simulink library "pixhawk_slib_swarm"  (R2022b)
settings: Solver=ode45  StartTime=0.0  StopTime=10.0  RelTol=1e-3
libraries: $bdroot x3, etargetslib x2, simulink x2
(part 1 of 2)
settings Model: Creator=skuznick  LastModifiedBy=童俊豪
settings SolverCC: AlgebraicLoopSolver=TrustRegion
settings DataIOCC: LimitDataPoints=on  SaveFormat=Array  ReturnWorkspaceOutputs=off
settings OptimizationCC: BlockReduction=off  BooleanDataType=off  LifeSpan=inf
settings DebuggingCC: SaveWithParameterizedLinksMsg=none  UnderspecifiedInitializationDetection=Classic  MergeDetectMultiDrivingBlocksExec=none  SignalResolutionControl=TryResolveAllWithWarning  UnconnectedInputMsg=warning  UnconnectedOutputMsg=warning  UnconnectedLineMsg=warning  AllowSymbolicDim=off  SFUnexpectedBacktrackingDiag=warning  SFNoUnconditionalDefaultTransitionDiag=warning  SFExecutionAtInitializationDiag=none  SFMachineParentedDataDiag=warning  ArithmeticOperatorsInVariantConditions=warning
settings HardwareCC: ProdBitPerPointer=32  ProdBitPerSizeT=32  ProdBitPerPtrDiffT=32  ProdLargestAtomicFloat=None  ProdIntDivRoundTo=Undefined  ProdEndianess=Unspecified  ProdWordSize=32  ProdHWDeviceType=32-bit Generic  TargetUnknown=on
settings ModelReferenceCC: EnableRefExpFcnMdlSchedulingChecks=on  PropagateSignalLabelsOutOfModel=off
settings SFSimCC: SimUseLocalCustomCode=off  CustomCodeUndefinedFunction=UseInterfaceOnly
settings RTWCC: RTWUseLocalCustomCode=off
settings CodeAppCC: StateflowObjectComments=on
settings GRTTargetCC: TargetLangStandard=C89/C90 (ANSI)
settings ConfigComp: CovMetricSettings=dw  CovSaveCumulativeToWorkspaceVar=on  CovSaveSingleToWorkspaceVar=on  CovExternalEMLEnable=off  CovSFcnEnable=off

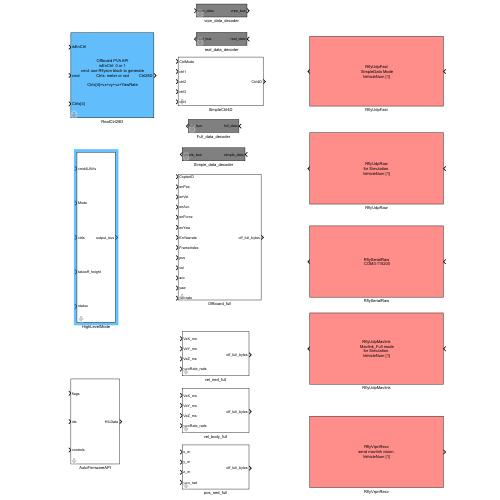
[thumbnail: Simulink's stored preview of the top-level diagram]
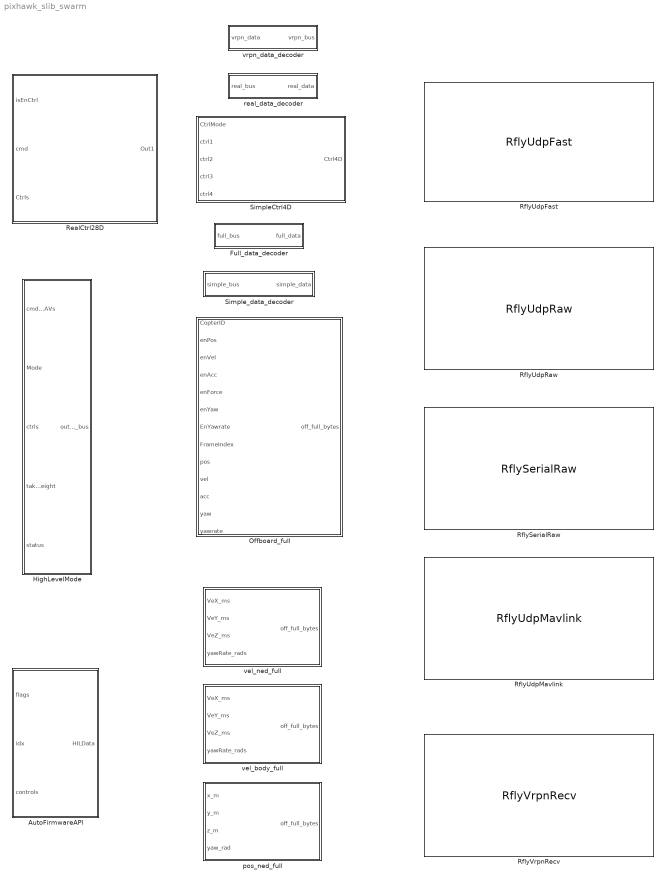
== system pixhawk_slib_swarm ==
  AutoFirmwareAPI : Subsystem  mask(AutoFirmwareAPI){}
      mask help:
      | This model is designed to generate 28 dims data for uav control with auto generated PX4  firmware by MATLAB.
      | The input data is to describe hil_actuator_controls, which has following meanings:
      | flags--user defined,  just keep sending and parsing consistent.
      | idx--for support more information, idx=0, treated as rfly_ctrl; idx=1, treated as rfly_ctrl1;idx=2, treated as rfly_ctrl2.
      | controls--detail imformation,can be control law or obstacle imformation.
      mask Help: eval('sharedhelp(''AutoFirmwareAPI'')');
  Full_data_decoder : Subsystem
      mask Help: eval('sharedhelp(''Full_data_decoder'')');
      mask DialogControl Control2 Prompt: (Add text here)
  HighLevelMode : Subsystem
      mask help:
      | Mode Control.
      |
      | 1 cmdUAVs should generate by "offical RflySim team" cmdUAVs "Rotary Switch".
      | 2   Mode will be explained as follows:
      |     Mode==1, x+y+z+yaw
      |     Mode==2, vx+vy+vz+yawrate
      |     Mode==3, accx+accy+accz+yawrate
      |     others, not supported
      | 3 ctrls only use first 4 elements and is described in local NED frame.
      | 4 takeoff_height, takeoff height.
      | 5 status means whether self check is passed, if not use, set true. Nothing will be send when status==false.
      mask Help: eval('sharedhelp(''HighLevelMode'')');
  Offboard_full : Subsystem
      mask Help: eval('sharedhelp(''Offboard_full'')');
      mask DialogControl Control2 Prompt: (Add text here)
  RealCtrl28D : Subsystem  mask{isX=off, isY=off, isZ=off, isVx=on, isVy=on, isVz=on, isAx=off, isAy=off, isAz=off, isYaw=off, isYawRate=on, EnIdxList=[1], isRcc=off, isForce=off, SamTime=-1}
      mask prompts: isX "x"; isY "y"; isZ "z"; isVx "vx"; isVy "vy"; isVz "vz"; isAx "ax"; isAy "ay"; isAz "az"; isYaw "yaw"; isYawRate "yawrate"; EnIdxList "mapList"; isRcc "Simulate Rcc Direct"; isForce "Enable Force"; SamTime "Sample Time (s)"
      mask help:
      | You can check the channels and prepare an input signal Ctrls with dimension and sequence corresponding to the of the checked channels.
      |
      | This Block enable offboard control for x y z vx vy vz ax ay az yaw yawrate，and support simulated Rcc direct control.
      |
      | # NED local world frame
      | x,y,z: position # in meters
      | Vx,Vy,Vz: velocity # in meters/second
      | Ax,Ay,Az: acceleration # in meters/second^2
      | yaw: euler angle of desired attitude in radians -PI..+PI
      | yawspeed: angular velocity around NED frame z-axis in radians/second
      |
      | In configuration page:
      | If "Simulate Rcc Direct" is checked, the module will send rcc signals to vehicle,  with relationship [vx, vy, vz, yawrate]->[ch1, ch2, ch3, ch4]. The user's [vx, vy, vz, yawrate] just in range [-1, 1], the block will map it to [1000-2000] automatically.
      | If "Enable Force" is checked, [ax, ay, az] will be treated as force.
      mask init:
      | SamTime=double(SamTime);
      mask Help: eval('sharedhelp(''RealCtrl28D'')');
      mask DialogControl Control2 Prompt: Select channels to control
      mask DialogControl Container3 Prompt: Option Functions
      mask Display:
      | nameList=["x";"y";"z";"vx";"vy";"vz";"ax";"ay";"az";"Yaw";"YawRate"];
      | nameList2=["isX";"isY";"isZ";"isVx";"isVy";"isVz";"isAx";"isAy";"isAz";"isYaw";"isYawRate"];
      | 
      | idx=0;
      | DispName='';
      | for i=1:length(nameList2)
      |     str0=char(nameList2(i));
      |     if strcmp(get_param(gcb,str0),'on') == true
      |         idx=idx+1;
      |         if idx==1
      |             DispName=[DispName,'',char(nameList(i))];
      |         else
      |             DispName=[DispName,'+',char(nameList(i))];
      |         end
      | 
      |         if mod(idx,4)==0
      |             DispName=[DispName,'\n'];
      |         end
      |     end
      | end
      | 
      | 
      | port_label('input', 1, 'isEnCtrl');
      | port_label('input', 2, 'cmd');
      | port_label('input', 3, ['Ctrls[',num2str(idx),']']);
      | port_label('output', 1, 'Ctrl28D');
      | 
      | fprintf(['Offboard PVA API\n isEnCtrl: 0 or 1 \n cmd: use Rflysim block to generate \n Ctrls: meter or rad \n\n','Ctrls[',num2str(idx),']=',DispName]);
      | 
      | set_param([gcb,'/isEnCtrl'],'PortDimensions',num2str(1));
      | set_param([gcb,'/cmd'],'PortDimensions',num2str(1));
      | set_param([gcb,'/Ctrls'],'PortDimensions',num2str(idx));
      | %set_param([gcb,'/OffboardAdvCtrlAPI'],'PortDimensions',num2str(idx));
  RflySerialRaw : S-Function  FunctionName=RflySerialRaw  Parameters=portname,baud,T  SFunctionDeploymentMode=off  EnableBusSupport=off  mask(RflySerialFast API){portname=COM3, baud=115200, T=1/30}
      mask prompts: portname "SerialPortName:"; baud "Baudrate or list (e.g., [57600,115200])"; T "Sample Time"
      mask help:
      | This block receives bytes from an serial connection.
      | 1. SerialPortName: Input the name of one pixhawk COM or multiple pixhawk COMs seperated by ','. For example, COM3 or COM3,COM4,COM5
      | 2. SelectAvailablePort: Prompt a window to select one or multiple COM port name
      | 3. baudrate or list: input the buadrate of all COMs or use a list to specify baudrate of each COM.
      |
      | input&output: variable-length unit_8 vector data from or to serial buffer.
      mask init:
      | if strcmp(computer(), 'PCWIN64')
      |     if isnumeric(portname)
      |         if portname>=10
      |             portname=['\\.\COM'+num2str(portname)];
      |         else
      |             portname=['COM'+num2str(portname)];
      |         end
      |     else
      |         dd=strsplit(portname,',');
      |         namestr='';
      |         for i=1:length(dd)
      |             name=strtrim(dd{1,i});
      |             if ~isempty(str2num(name))
      |                 nNnum=str2double(name);
      |                 if nNnum>=10
      |                     name=['\\.\COM'+num2str(nNnum)];
      |                 else
      |                     name=['COM'+num2str(nNnum)];
      |                 end
      |             end
      |             
      |         
      |             if length(name)>4
      |                 name=['\\.\',name];
      |             end
      |         
      |             namestr=[namestr,name];
      |             if i~=length(dd)
      |                 namestr=[namestr,','];
      |             end
      |         end
      |         portname=namestr;
      |     end
      | end
      mask Help: eval('sharedhelp(''RflySerialRaw'')');
      mask DialogControl Control3 Prompt: SelectAvailablePort
      mask DialogControl Control3 Callback:
      | portList = seriallist;
      | if ~isempty(portList)
      |     CellTmp={};
      |     for i=1:length(portList)
      |         CellTmp{i,1}=char(portList(i));
      |     end
      |     [indx,tf] = listdlg('ListString',CellTmp,'ListSize',[160,100]);
      |     if tf
      |         maskObj = Simulink.Mask.get(gcb);
      |         for i=1:length(maskObj.Parameters)
      |             if strcmp(maskObj.Parameters(i).Name,'portname')
      |                 myStr='';
      |                 for j=1:length(indx)
      |                     myStr=[myStr,CellTmp{indx(j),1}];
      |                     if j~=length(indx)
      |                         myStr=[myStr,','];
      |                     end
      |                 end
      |                 %maskObj.Parameters(i).set('Value',myStr);
      |                 maskObj.Parameters(i).Value=myStr;
      |             end
      |         end
      | 
      |     end
      | else
      |     msgbox('No avaliable COM port.')
      | end
      mask Display: fprintf(['RflySerialRaw\n ',get_param(gcb,'portname'),':',get_param(gcb,'baud')]);
  RflyUdpFast : S-Function  FunctionName=RflyUdpFast  Parameters=idx,num,modeValue,T,ip,Gps,port,isSame  SFunctionDeploymentMode=off  EnableBusSupport=off  mask(RflyUdpFast API){ip=127.0.0.1, idx=1, num=1, mode=SimpleData Mode, Gps=[40.1540302,116.2593683,50.0], port=20100, isSame=off, T=1/30, modeValue=0}
      mask prompts: ip "Target IP Address"; idx "Start CopterID"; num "Vehicle number or CopterID list (e.g., [1 3 4])"; mode "UDP Mode"; Gps "GPS Orin [Lat Lon (degree) Alt(m)] for GlobalPos"; port "Base UDP Port (for CopterID#1)"; isSame "useSamePort"; T "Sample Time"
      mask help:
      | RflySimAPIs for multiple uav data acquire and control
      | 1. Target IP: The IP of PC running CopterSims to receive data
      | 2. Vehicle number: Total vehicle number with StartID=1.
      | For example Vehicle number=3 for a CopterID list [1 2 3]
      | 3. CopterID List: a vector of CopterIDs, like [1 2 3] or [1:3] or [4 5 7]
      | 4. UDP Mode: Full or simple mode to transmit data
      | 5. GPS Orin: the lat lon alt of GPS position for calculate global position
      | 6. check the "Help" button for the definition
      mask init:
      | if strcmp(mode,'FullData Mode')
      |     modeValue = 0;
      | elseif strcmp(mode,'SimpleData Mode') 
      |     modeValue = 1;
      | elseif strcmp(mode,'UltraSimple Mode') 
      |     modeValue = 2;
      | else
      |     modeValue = 0;
      | end
      | 
      | if length(num)==1
      |     if str2double(get_param(gcb,'num')) == num
      |         num = 1:num;
      |     end
      | end
      mask Help: eval('sharedhelp(''RflyUdpFast'')');
      mask TypeOptions mode: FullData Mode | SimpleData Mode
      mask Display:
      | numstr=get_param(gcb,'num');
      | if strcmp(numstr,'1')
      |     numstr='[1]';
      | end
      | fprintf(['RflyUdpFast\n ',get_param(gcb,'mode'),'\nVehicleNum ',numstr]);
  RflyUdpMavlink : S-Function  FunctionName=RflyUdpMavlink  Parameters=idx,num,ip,T,port,isSame,Gps,udpmode  SFunctionDeploymentMode=off  EnableBusSupport=off  mask(RflyUdpReal API){idx=1, ip1=127.0.0.1, ip=192.168.31.101, num=1, port=15501, Gps=[40.1540302,116.2593683,50.0], udpmode=Mavlink_Full, T=1/30, isSame=off}
      mask prompts: idx "Start Index"; ip1 "Target IP Address"; ip "Base IP Address or IP list seperated by ','"; num "Vehicle number or CopterID list (e.g., [1 3 4])"; port "Base UDP Port or list"; Gps "GPS Orin [Lat Lon (degree) Alt(m)] for GlobalPos"; udpmode "Udp Mode"; T "Sample Time"; isSame "RealflyMode"
      mask help:
      | RflySimAPIs for multiple real uav data acquire and control
      | 1. Base IP: The bash IP of the first UAV to receive MAVLink data
      | 2. IP list: a string like 191.168.151.101,191.168.151.102 to specify the ip of each UAV
      | 3. Vehicle number: Total vehicle number with StartID=1.
      | For example Vehicle number=3 for a CopterID list [1 2 3]
      | 4. CopterID List: a vector of CopterIDs, like [1 2 3] or [1:3] or [4 5 7]
      | 5. Base UDP Port: The base port of the first UAV's mavlink port. You can also use a port list to specify the port of each UAV
      | 6. RealflyMode: Checked for real uav control, the IP and port will auto increase 1 according to CopterID increase.
      | Not checked for RflySim UDP simulation, the IP will not change and the port will +2 for each CopterID.
      |
      | Input and output char arrays from buf for mavlink encode and decoder
      mask init:
      | if isSame<0.5
      |     ip=ip1;
      | end
      | 
      | if length(num)==1
      |     if str2double(get_param(gcb,'num')) == num
      |         num = 1:num;
      |     end
      | end
      mask Help: eval('sharedhelp(''RflyUdpMavlink'')');
      mask TypeOptions udpmode: Mavlink_Full | Mavlink_Simp | Mavlink_Real
      mask Callback isSame:
      | maskObj = Simulink.Mask.get(gcb);
      | for i=1:length(maskObj.Parameters)
      |     if strcmp(maskObj.Parameters(i).Name,'Gps')
      |         if strcmp(get_param(gcb,'isSame'),'off')
      |             if strcmp(maskObj.Parameters(i).Enabled,'off')
      |                 maskObj.Parameters(i).Enabled='on';
      |                 maskObj.Parameters(i).Visible='on';
      |             end
      |         else
      |             if strcmp(maskObj.Parameters(i).Enabled,'on')
      |                 maskObj.Parameters(i).Enabled='off';
      |                 maskObj.Parameters(i).Visible='off';
      |             end
      |         end
      |     end
      | end
      | for i=1:length(maskObj.Parameters)
      |     if strcmp(maskObj.Parameters(i).Name,'port')
      |         if strcmp(get_param(gcb,'isSame'),'off')
      |             if strcmp(maskObj.Parameters(i).Enabled,'on')
      |                 maskObj.Parameters(i).Enabled='off';
      |                 maskObj.Parameters(i).Visible='off';
      |             end
      |         else
      |             if strcmp(maskObj.Parameters(i).Enabled,'off')
      |                 maskObj.Parameters(i).Enabled='on';
      |                 maskObj.Parameters(i).Visible='on';
      |             end
      |         end
      |     end
      | end
      | for i=1:length(maskObj.Parameters)
      |     if strcmp(maskObj.Parameters(i).Name,'ip1')
      |         if strcmp(get_param(gcb,'isSame'),'on')
      |             if strcmp(maskObj.Parameters(i).Enabled,'on')
      |                 maskObj.Parameters(i).Enabled='off';
      |                 maskObj.Parameters(i).Visible='off';
      |             end
      |         else
      |             if strcmp(maskObj.Parameters(i).Enabled,'off')
      |                 maskObj.Parameters(i).Enabled='on';
      |                 maskObj.Parameters(i).Visible='on';
      |             end
      |         end
      |     end
      | end
      | for i=1:length(maskObj.Parameters)
      |     if strcmp(maskObj.Parameters(i).Name,'ip')
      |         if strcmp(get_param(gcb,'isSame'),'on')
      |             if strcmp(maskObj.Parameters(i).Enabled,'off')
      |                 maskObj.Parameters(i).Enabled='on';
      |                 maskObj.Parameters(i).Visible='on';
      |             end
      |         else
      |             if strcmp(maskObj.Parameters(i).Enabled,'on')
      |                 maskObj.Parameters(i).Enabled='off';
      |                 maskObj.Parameters(i).Visible='off';
      |             end
      |         end
      |     end
      | end
      | 
      | for i=1:length(maskObj.Parameters)
      |     if strcmp(maskObj.Parameters(i).Name,'udpmode')
      |         if strcmp(get_param(gcb,'isSame'),'off')
      |             if strcmp(maskObj.Parameters(i).Enabled,'off')
      |                 maskObj.Parameters(i).Enabled='on';
      |                 maskObj.Parameters(i).Visible='on';
      |             end
      |         else
      |             if strcmp(maskObj.Parameters(i).Enabled,'on')
      |                 maskObj.Parameters(i).Enabled='off';
      |                 maskObj.Parameters(i).Visible='off';
      |             end
      |         end
      |     end
      | end
      mask Display:
      | myname='for Simulation.';
      | if strcmp(get_param(gcb,'isSame'),'on')
      |     myname='for Real fly.';
      | end
      | numstr=get_param(gcb,'num');
      | if strcmp(numstr,'1')
      |     numstr='[1]';
      | end
      | fprintf(['RflyUdpMavlink\n ',get_param(gcb,'udpmode'),' mode\n',myname,'\nVehicleNum ',numstr]);
  RflyUdpRaw : S-Function  FunctionName=RflyUdpRaw  Parameters=idx,num,ip,T,port,isSame  SFunctionDeploymentMode=off  EnableBusSupport=off  mask(RflyUdpReal API){idx=1, ip1=127.0.0.1, ip=192.168.31.101, num=1, port=15501, T=1/30, isSame=off}
      mask prompts: idx "Start Index"; ip1 "Target IP Address"; ip "Base IP Address or IP list seperated by ','"; num "Vehicle number or CopterID list (e.g., [1 3 4])"; port "Base UDP Port or list"; T "Sample Time"; isSame "RealflyMode"
      mask help:
      | RflySimAPIs for multiple real uav data acquire and control
      | 1. IP Address: The bash IP of the first UAV to receive MAVLink data (127.0.0.1 for Simulation or remote ip for real fly)
      | 2. IP list: a string like 191.168.151.101,191.168.151.102 to specify the ip of each UAV
      | 3. Vehicle number: Total vehicle number with StartID=1.
      | For example Vehicle number=3 for a CopterID list [1 2 3]
      | 4. CopterID List: a vector of CopterIDs, like [1 2 3] or [1:3] or [4 5 7]
      | 5. Base UDP Port: The base port of the first UAV's mavlink port. You can also use a port list to specify the port of each UAV
      | 6. RealflyMode: Checked for real uav control, the IP and port will auto increase 1 according to CopterID increase.
      | Not checked for RflySim UDP simulation, the IP will not change and the port will +2 for each CopterID.
      |
      | Input and output char arrays from buf for mavlink encode and decoder
      mask init:
      | if isSame<0.5
      |     ip=ip1;
      | end
      | 
      | if length(num)==1
      |     if str2double(get_param(gcb,'num')) == num
      |         num = 1:num;
      |     end
      | end
      mask Help: eval('sharedhelp(''RflyUdpRaw'')');
      mask Callback isSame:
      | maskObj = Simulink.Mask.get(gcb);
      | for i=1:length(maskObj.Parameters)
      |     if strcmp(maskObj.Parameters(i).Name,'port')
      |         if strcmp(get_param(gcb,'isSame'),'off')
      |             maskObj.Parameters(i).Enabled='off';
      |             maskObj.Parameters(i).Visible='off';
      |         else
      |             maskObj.Parameters(i).Enabled='on';
      |             maskObj.Parameters(i).Visible='on';
      |         end
      |     end
      | end
      | for i=1:length(maskObj.Parameters)
      |     if strcmp(maskObj.Parameters(i).Name,'ip1')
      |         if strcmp(get_param(gcb,'isSame'),'on')
      |             maskObj.Parameters(i).Enabled='off';
      |             maskObj.Parameters(i).Visible='off';
      |         else
      |             maskObj.Parameters(i).Enabled='on';
      |             maskObj.Parameters(i).Visible='on';
      |         end
      |     end
      | end
      | for i=1:length(maskObj.Parameters)
      |     if strcmp(maskObj.Parameters(i).Name,'ip')
      |         if strcmp(get_param(gcb,'isSame'),'on')
      |             maskObj.Parameters(i).Enabled='on';
      |             maskObj.Parameters(i).Visible='on';
      |         else
      |             maskObj.Parameters(i).Enabled='off';
      |             maskObj.Parameters(i).Visible='off';
      |         end
      |     end
      | end
      mask Display:
      | myname='for Simulation.';
      | if strcmp(get_param(gcb,'isSame'),'on')
      |     myname='for Real fly.';
      | end
      | numstr=get_param(gcb,'num');
      | if strcmp(numstr,'1')
      |     numstr='[1]';
      | end
      | fprintf(['RflyUdpRaw\n',myname,'\nVehicleNum ',numstr]);
  RflyVrpnRecv : S-Function  FunctionName=RflyVrpnRecv  Parameters=vrpn_ip,num,T,isSend,drone_ip,drone_port,vrScaleX,vrScaleY,vrScaleZ  SFunctionDeploymentMode=off  EnableBusSupport=off  mask(RflyUdpReal API){vrpn_ip=127.0.0.1, num=1, T=1/30, isSend=on, drone_ip=192.168.151.101, drone_port=15501, vrScaleX=1.0, vrScaleY=1.0, vrScaleZ=1.0}
      mask prompts: vrpn_ip "Vrpn IP Address"; num "Vehicle number or CopterID list (e.g., [1 3 4])"; T "Sample Time"; isSend "isSendVision"; drone_ip "Drone base IP Address or IP list seperated by ','"; drone_port "Drone base UDP Port or list"; vrScaleX "VR Scale X"; vrScaleY "Y"; vrScaleZ "Z"
      mask help:
      | RflySimAPIs for multiple real uav data acquire and control
      | 1. Base IP: The bash IP of the first UAV to receive MAVLink data
      | 2. IP list: a string like 191.168.151.101,191.168.151.102 to specify the ip of each UAV
      | 3. Vehicle number: Total vehicle number with StartID=1.
      | For example Vehicle number=3 for a CopterID list [1 2 3]
      | 4. CopterID List: a vector of CopterIDs, like [1 2 3] or [1:3] or [4 5 7]
      | 5. Base UDP Port: The base port of the first UAV's mavlink port. You can also use a port list to specify the port of each UAV
      | 6. RealflyMode: Checked for real uav control, the IP and port will auto increase 1 according to CopterID increase.
      | 7.Scale for combination of virtual and real elements for X direction.
      | 8.Scale for combination of virtual and real elements for Y direction.
      | 9.Scale for combination of virtual and real elements for vertical direction.
      | Not checked for RflySim UDP simulation, the IP will not change and the port will +2 for each CopterID.
      |
      | Input and output char arrays from buf for mavlink encode and decoder
      mask init:
      | if length(num)==1
      |     if str2double(get_param(gcb,'num')) == num
      |         num = 1:num;
      |     end
      | end
      mask Help: eval('sharedhelp(''RflyVrpnRecv'')');
      mask Callback isSend:
      | maskObj = Simulink.Mask.get(gcb);
      | for i=1:length(maskObj.Parameters)
      |     if strcmp(maskObj.Parameters(i).Name,'drone_ip')
      |         if strcmp(get_param(gcb,'isSend'),'on')
      |             if strcmp(maskObj.Parameters(i).Enabled,'off')
      |                 maskObj.Parameters(i).Enabled='on';
      |                 maskObj.Parameters(i).Visible='on';
      |             end
      |         else
      |             if strcmp(maskObj.Parameters(i).Enabled,'on')
      |                 maskObj.Parameters(i).Enabled='off';
      |                 maskObj.Parameters(i).Visible='off';
      |             end
      |         end
      |     end
      | end
      | for i=1:length(maskObj.Parameters)
      |     if strcmp(maskObj.Parameters(i).Name,'drone_port')
      |         if strcmp(get_param(gcb,'isSend'),'on')
      |             if strcmp(maskObj.Parameters(i).Enabled,'off')
      |                 maskObj.Parameters(i).Enabled='on';
      |                 maskObj.Parameters(i).Visible='on';
      |             end
      |         else
      |             if strcmp(maskObj.Parameters(i).Enabled,'on')
      |                 maskObj.Parameters(i).Enabled='off';
      |                 maskObj.Parameters(i).Visible='off';
      |             end
      |         end
      |     end
      | end
      mask Display:
      | myname='not send vision.';
      | if strcmp(get_param(gcb,'isSend'),'on')
      |     myname='send mavlink vision.';
      | end
      | numstr=get_param(gcb,'num');
      | if strcmp(numstr,'1')
      |     numstr='[1]';
      | end
      | fprintf(['RflyVrpnRecv\n',myname,'\nVehicleNum ',numstr]);
  SimpleCtrl4D : Subsystem
      mask Help: eval('sharedhelp(''SimpleCtrl4D'')');
      mask DialogControl Control2 Prompt: (Add text here)
  Simple_data_decoder : Subsystem
      mask Help: eval('sharedhelp(''Simple_data_decoder'')');
      mask DialogControl Control2 Prompt: (Add text here)
  pos_ned_full : Subsystem
      mask Help: eval('sharedhelp(''pos_ned_full'')');
      mask DialogControl Control2 Prompt: (Add text here)
  real_data_decoder : Subsystem
      mask Help: eval('sharedhelp(''real_data_decoder'')');
      mask DialogControl Control2 Prompt: (Add text here)
  vel_body_full : Subsystem
      mask Help: eval('sharedhelp(''vel_body_full'')');
      mask DialogControl Control2 Prompt: (Add text here)
  vel_ned_full : Subsystem
      mask Help: eval('sharedhelp(''vel_ned_full'')');
      mask DialogControl Control2 Prompt: (Add text here)
  vrpn_data_decoder : Subsystem
      mask Help: eval('sharedhelp(''vrpn_data_decoder'')');
      mask DialogControl Control2 Prompt: (Add text here)

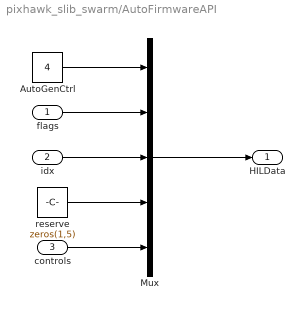
== system pixhawk_slib_swarm/AutoFirmwareAPI ==
  flags : Inport
  idx : Inport  Port=2
  controls : Inport  Port=3
  AutoGenCtrl : Constant  Value=4
  Mux : Mux  Inputs=5
  reserve : Constant  Value=zeros(1,5)
  HILData : Outport  VectorParamsAs1DForOutWhenUnconnected=off
  wires:
  Mux/1 -> HILData/1
  flags/1 -> Mux/2
  idx/1 -> Mux/3
  controls/1 -> Mux/5
  AutoGenCtrl/1 -> Mux/1
  reserve/1 -> Mux/4

== system pixhawk_slib_swarm/Full_data_decoder ==
  note: AngEular
  note: localVel
  note: localPos
  full_data : Inport
  Bus Creator : BusCreator  Inputs=17
  Decoder1 : MATLAB Function  TreatAsAtomicUnit=on
  full_bus : Outport  VectorParamsAs1DForOutWhenUnconnected=off
  wires:
  Decoder1/17(resrveFloat) -> Bus Creator/17  "resrveFloat"
  Decoder1/1(globalPos) -> Bus Creator/1  "globalPos"
  Decoder1/7(gpsHome) -> Bus Creator/7  "gpsHome"
  Decoder1/12(satellites_visible) -> Bus Creator/12  "satellites_visible"
  Bus Creator/1 -> full_bus/1
  full_data/1 -> Decoder1/1(u)
  Decoder1/14(resrveInit) -> Bus Creator/14  "resrveInit"
  Decoder1/13(fix_type) -> Bus Creator/13  "fix_type"
  Decoder1/15(pos_horiz_accuracy) -> Bus Creator/15  "pos_horiz_accuracy"
  Decoder1/16(pos_vert_accuracy) -> Bus Creator/16
  Decoder1/9(copterID) -> Bus Creator/9  "copterID"
  Decoder1/10(relative_alt) -> Bus Creator/10  "relative_alt"
  Decoder1/11(hdg) -> Bus Creator/11  "hdg"
  Decoder1/8(time_boot_ms) -> Bus Creator/8  "time_boot_ms"
  Decoder1/6(GpsVel) -> Bus Creator/6  "GpsVel"
  Decoder1/5(GpsPos) -> Bus Creator/5  "GpsPos"
  Decoder1/2(AngEular) -> Bus Creator/2  "AngEular"
  Decoder1/3(localPos) -> Bus Creator/3  "localPos"
  Decoder1/4(localVel) -> Bus Creator/4  "localVel"

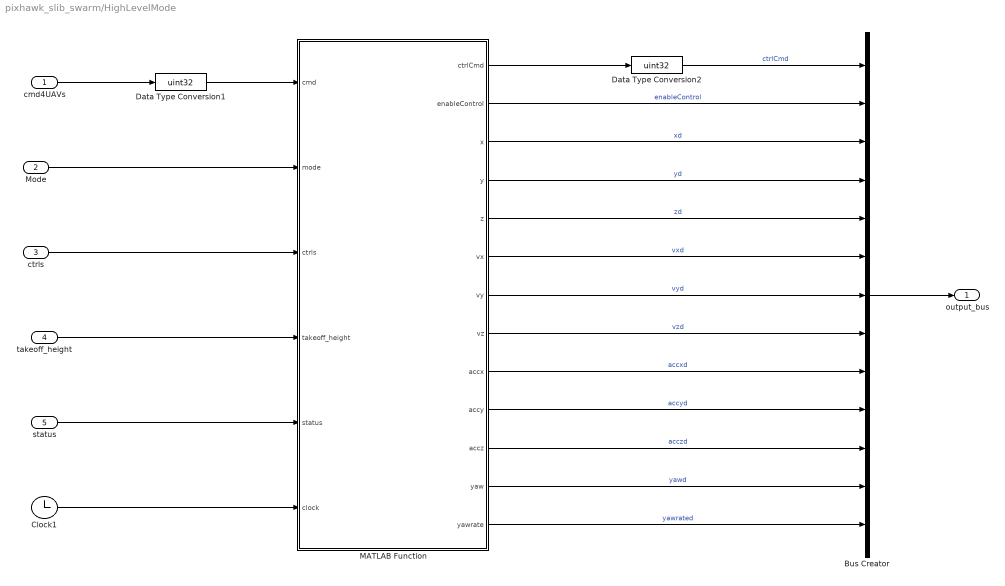
== system pixhawk_slib_swarm/HighLevelMode ==
  cmd4UAVs : Inport
  Mode : Inport  Port=2  PortDimensions=1
  ctrls : Inport  Port=3  PortDimensions=16
  takeoff_height : Inport  Port=4
  status : Inport  Port=5
  Bus Creator : BusCreator  Inputs=13
  Clock1 : Clock
  Data Type Conversion1 : DataTypeConversion  OutDataTypeStr=uint32  SaturateOnIntegerOverflow=off  RndMeth=Floor
  Data Type Conversion2 : DataTypeConversion  OutDataTypeStr=uint32  SaturateOnIntegerOverflow=off  RndMeth=Floor
  MATLAB Function : MATLAB Function  TreatAsAtomicUnit=on
  output_bus : Outport  VectorParamsAs1DForOutWhenUnconnected=off
  wires:
  cmd4UAVs/1 -> Data Type Conversion1/1
  Data Type Conversion1/1 -> MATLAB Function/1(cmd)
  Clock1/1 -> MATLAB Function/6(clock)
  status/1 -> MATLAB Function/5(status)
  MATLAB Function/1(ctrlCmd) -> Data Type Conversion2/1
  Data Type Conversion2/1 -> Bus Creator/1  "ctrlCmd"
  MATLAB Function/2(enableControl) -> Bus Creator/2  "enableControl"
  MATLAB Function/3(x) -> Bus Creator/3  "xd"
  MATLAB Function/4(y) -> Bus Creator/4  "yd"
  MATLAB Function/5(z) -> Bus Creator/5  "zd"
  MATLAB Function/6(vx) -> Bus Creator/6  "vxd"
  MATLAB Function/7(vy) -> Bus Creator/7  "vyd"
  MATLAB Function/8(vz) -> Bus Creator/8  "vzd"
  MATLAB Function/9(accx) -> Bus Creator/9  "accxd"
  MATLAB Function/10(accy) -> Bus Creator/10  "accyd"
  MATLAB Function/11(accz) -> Bus Creator/11  "acczd"
  MATLAB Function/12(yaw) -> Bus Creator/12  "yawd"
  MATLAB Function/13(yawrate) -> Bus Creator/13  "yawrated"
  ctrls/1 -> MATLAB Function/3(ctrls)
  Mode/1 -> MATLAB Function/2(mode)
  Bus Creator/1 -> output_bus/1
  takeoff_height/1 -> MATLAB Function/4(takeoff_height)

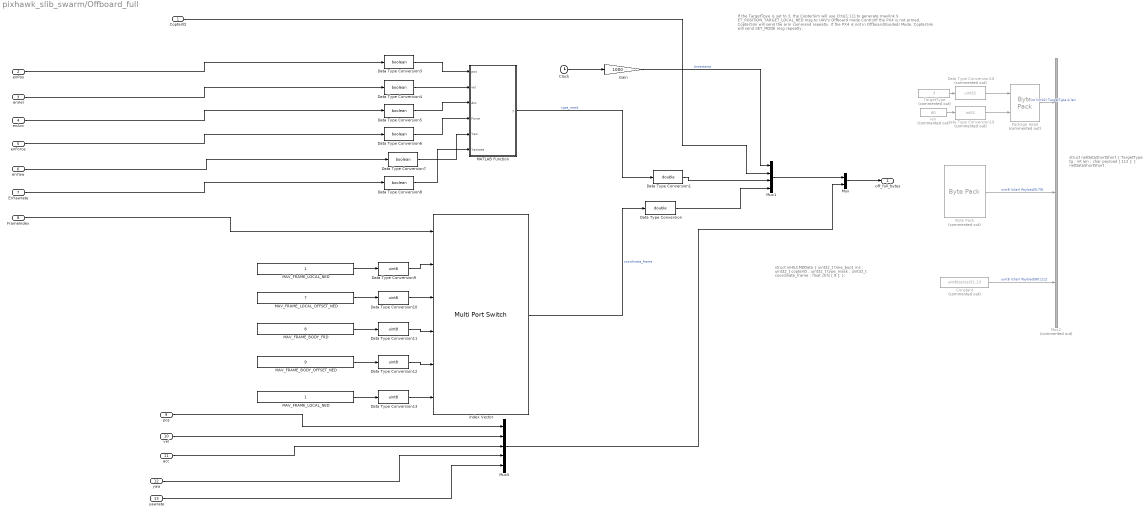
== system pixhawk_slib_swarm/Offboard_full ==
  note: struct netDataShortShort {
      | TargetType tg ;
      | int len ;
      | char payload [ 112 ];
      | } netDataShortShort ;
  note: struct inHILCMDData {
      | uint32_t time_boot_ms ;
      | uint32_t copterID ;
      | uint32_t type_mask ;
      | uint32_t coordinate_frame ;
      | float ctrls [ 9 ];
      | };
  note: If the TargetTpye is set to 3, the CopterSim will use Ctrs[1:11] to generate mavlink S ET_POSITION_TARGET_LOCAL_NED msg to UAV's Offboard mode Control，
      | If the PX4 is not armed, CopterSim will send the arm command repeatly. If the PX4 is not in Offboard(Guided) Mode, CopterSim will send SET_MODE msg repeatly.
  CopterID : Inport
  enPos : Inport  Port=2
  enVel : Inport  Port=3
  enAcc : Inport  Port=4
  enForce : Inport  Port=5
  enYaw : Inport  Port=6
  EnYawrate : Inport  Port=7
  FrameIndex : Inport  Port=8
  pos : Inport  Port=9  PortDimensions=3
  vel : Inport  Port=10  PortDimensions=3
  acc : Inport  Port=11  PortDimensions=3
  yaw : Inport  Port=12  PortDimensions=1
  yawrate : Inport  Port=13  PortDimensions=1
  Byte Pack : etargetslib/Byte Pack  Commented=on  datatypes={'uint32','single'}  byteAlign=1
  Clock : Clock
  Constant : Constant  Commented=on  Value=uint8(zeros(32,1))
  Data Type Conversion : DataTypeConversion  OutDataTypeStr=double  SaturateOnIntegerOverflow=off  RndMeth=Floor
  Data Type Conversion1 : DataTypeConversion  OutDataTypeStr=double  SaturateOnIntegerOverflow=off  RndMeth=Floor
  Data Type Conversion{9..13} (5 alike) : DataTypeConversion  OutDataTypeStr=uint8  SaturateOnIntegerOverflow=off  RndMeth=Floor
  Data Type Conversion18 : DataTypeConversion  Commented=on  OutDataTypeStr=uint32  SaturateOnIntegerOverflow=off  RndMeth=Floor
  Data Type Conversion19 : DataTypeConversion  Commented=on  OutDataTypeStr=int32  SaturateOnIntegerOverflow=off  RndMeth=Floor
  Data Type Conversion{3..8} (6 alike) : DataTypeConversion  OutDataTypeStr=boolean  SaturateOnIntegerOverflow=off  RndMeth=Floor
  Gain : Gain  Gain=1000
  Index Vector : MultiPortSwitch  DataPortOrder=Zero-based contiguous  Inputs=5  zeroidx=on  SaturateOnIntegerOverflow=off  InputSameDT=off
  MATLAB Function : MATLAB Function  TreatAsAtomicUnit=on
  MAV_FRAME_BODY_FRD : Constant  Value=8
  "MAV_FRAME_BODY_OFFSET_NED " : Constant  Value=9
  MAV_FRAME_LOCAL_NED : Constant
  "MAV_FRAME_LOCAL_NED " : Constant
  MAV_FRAME_LOCAL_OFFSET_NED : Constant  Value=7
  Mux : Mux  Inputs=2
  Mux1 : Mux
  Mux2 : Mux  Commented=on  Inputs=3
  Mux5 : Mux  Inputs=5
  Package Head : etargetslib/Byte Pack  Commented=on  datatypes={'uint32','int32'}  byteAlign=4
  TargetType : Constant  Commented=on  Value=3  OutDataTypeStr=Inherit: Inherit via back propagation
  len : Constant  Commented=on  Value=80  OutDataTypeStr=Inherit: Inherit via back propagation
  off_full_bytes : Outport
  wires:
  Data Type Conversion7/1 -> MATLAB Function/5(Yaw)
  Data Type Conversion6/1 -> MATLAB Function/4(Force)
  vel/1 -> Mux5/2
  MAV_FRAME_BODY_FRD/1 -> Data Type Conversion11/1
  Data Type Conversion3/1 -> MATLAB Function/1(pos)
  Data Type Conversion5/1 -> MATLAB Function/3(Acc)
  Data Type Conversion4/1 -> MATLAB Function/2(vel)
  Data Type Conversion8/1 -> MATLAB Function/6(Yawrate)
  enAcc/1 -> Data Type Conversion5/1
  enYaw/1 -> Data Type Conversion7/1
  EnYawrate/1 -> Data Type Conversion8/1
  enForce/1 -> Data Type Conversion6/1
  "MAV_FRAME_LOCAL_NED "/1 -> Data Type Conversion9/1
  enPos/1 -> Data Type Conversion3/1
  Data Type Conversion9/1 -> Index Vector/2
  Data Type Conversion10/1 -> Index Vector/3
  Index Vector/1 -> Data Type Conversion/1  "coordinate_frame"
  Constant/1 -> Mux2/3  "uint8 (char) Payload[80:111]"
  Data Type Conversion18/1 -> Package Head/1
  Clock/1 -> Gain/1
  len/1 -> Data Type Conversion19/1
  Mux5/1 -> Mux/2
  MATLAB Function/1(y) -> Data Type Conversion1/1  "type_mask"
  Package Head/1 -> Mux2/1  "int (int32) TargetType & len"
  TargetType/1 -> Data Type Conversion18/1
  Gain/1 -> Mux1/1  "timestamp"
  Data Type Conversion19/1 -> Package Head/2
  pos/1 -> Mux5/1
  Byte Pack/1 -> Mux2/2  "uint8 (char) Payload[0:79]"
  Data Type Conversion13/1 -> Index Vector/6
  Data Type Conversion12/1 -> Index Vector/5
  acc/1 -> Mux5/3
  FrameIndex/1 -> Index Vector/1
  MAV_FRAME_LOCAL_NED/1 -> Data Type Conversion13/1
  MAV_FRAME_LOCAL_OFFSET_NED/1 -> Data Type Conversion10/1
  Data Type Conversion11/1 -> Index Vector/4
  "MAV_FRAME_BODY_OFFSET_NED "/1 -> Data Type Conversion12/1
  enVel/1 -> Data Type Conversion4/1
  yaw/1 -> Mux5/4
  yawrate/1 -> Mux5/5
  CopterID/1 -> Mux1/2
  Mux1/1 -> Mux/1
  Mux/1 -> off_full_bytes/1
  Data Type Conversion/1 -> Mux1/4
  Data Type Conversion1/1 -> Mux1/3

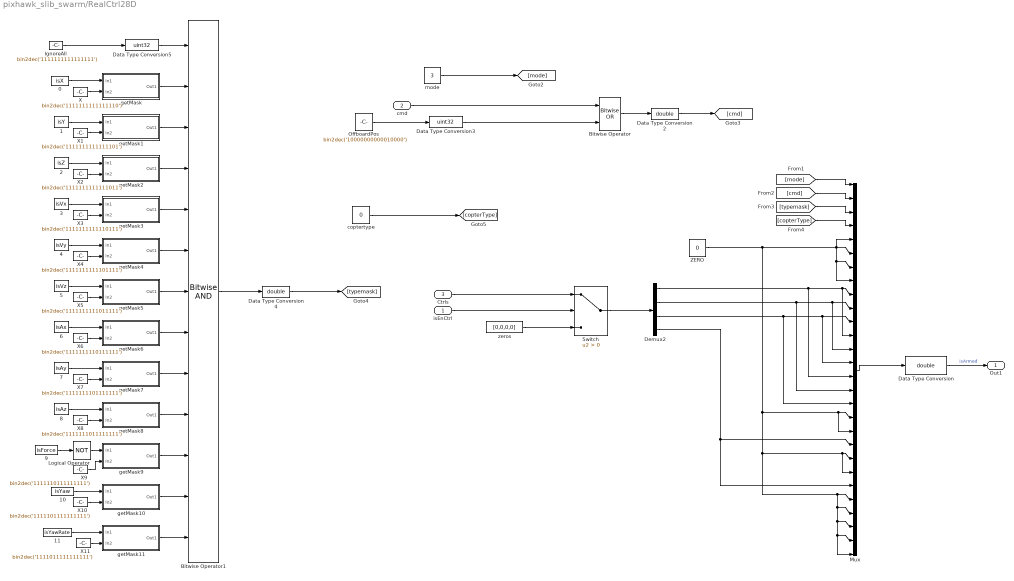
== system pixhawk_slib_swarm/RealCtrl28D ==
  isEnCtrl : Inport  PortDimensions=1
  cmd : Inport  Port=2  OutDataTypeStr=uint32  PortDimensions=1
  Ctrls : Inport  Port=3  PortDimensions=4
  0 : Constant  Value=isX
  1 : Constant  Value=isY
  10 : Constant  Value=isYaw
  11 : Constant  Value=isYawRate
  2 : Constant  Value=isZ
  3 : Constant  Value=isVx
  4 : Constant  Value=isVy
  5 : Constant  Value=isVz
  6 : Constant  Value=isAx
  7 : Constant  Value=isAy
  8 : Constant  Value=isAz
  9 : Constant  Value=isForce
  Bitwise Operator : simulink/Logic and Bit Operations/Bitwise Operator  logicop=OR  UseBitMask=off  NumInputPorts=2  BitMask=bin2dec('11011001')  BitMaskRealWorld=Stored Integer
  Bitwise Operator1 : simulink/Logic and Bit Operations/Bitwise Operator  logicop=AND  UseBitMask=off  NumInputPorts=13  BitMask=bin2dec('11011001')  BitMaskRealWorld=Stored Integer
  Data Type Conversion : DataTypeConversion  OutDataTypeStr=double  SaturateOnIntegerOverflow=off  RndMeth=Floor
  Data Type Conversion2 : DataTypeConversion  OutDataTypeStr=double  SaturateOnIntegerOverflow=off  RndMeth=Floor
  Data Type Conversion3 : DataTypeConversion  OutDataTypeStr=uint32  SaturateOnIntegerOverflow=off  RndMeth=Floor
  Data Type Conversion4 : DataTypeConversion  OutDataTypeStr=double  SaturateOnIntegerOverflow=off  RndMeth=Floor
  Data Type Conversion5 : DataTypeConversion  OutDataTypeStr=uint32  SaturateOnIntegerOverflow=off  RndMeth=Floor
  Demux2 : Demux
  IgnoreAll : Constant  Value=bin2dec('1111111111111111')
  Logical Operator : Logic  Operator=NOT  AllPortsSameDT=off  OutDataTypeStr=boolean
  Mux : Mux  Inputs=28
  OffboardPos : Constant  Value=bin2dec('10000000000010000')
  Switch : Switch  Criteria=u2 > Threshold  SaturateOnIntegerOverflow=off  InputSameDT=off
  X : Constant  Value=bin2dec('1111111111111110')
  X1 : Constant  Value=bin2dec('1111111111111101')
  X10 : Constant  Value=bin2dec('1111101111111111')
  X11 : Constant  Value=bin2dec('1111011111111111')
  X2 : Constant  Value=bin2dec('1111111111111011')
  X3 : Constant  Value=bin2dec('1111111111110111')
  X4 : Constant  Value=bin2dec('1111111111101111')
  X5 : Constant  Value=bin2dec('1111111111011111')
  X6 : Constant  Value=bin2dec('1111111110111111')
  X7 : Constant  Value=bin2dec('1111111101111111')
  X8 : Constant  Value=bin2dec('1111111011111111')
  X9 : Constant  Value=bin2dec('1111110111111111')
  ZERO : Constant  Value=0
  coptertype : Constant  Value=0
  getMask : Subsystem
  getMask1 : Subsystem
  getMask10 : Subsystem
  getMask11 : Subsystem
  getMask2 : Subsystem
  getMask3 : Subsystem
  getMask4 : Subsystem
  getMask5 : Subsystem
  getMask6 : Subsystem
  getMask7 : Subsystem
  getMask8 : Subsystem
  getMask9 : Subsystem
  mode : Constant  Value=3
  zeros : Constant  Value=[0,0,0,0]
  Out1 : Outport  VectorParamsAs1DForOutWhenUnconnected=off
  wires:
  Data Type Conversion/1 -> Out1/1  "isArmed"
  Data Type Conversion5/1 -> Bitwise Operator1/1
  getMask/1(Out1) -> Bitwise Operator1/2
  Bitwise Operator1/1 -> Data Type Conversion4/1
  Data Type Conversion3/1 -> Bitwise Operator/2
  Bitwise Operator/1 -> Data Type Conversion2/1
  OffboardPos/1 -> Data Type Conversion3/1
  Mux/1 -> Data Type Conversion/1
  IgnoreAll/1 -> Data Type Conversion5/1
  mode/1 -> [mode]
  Data Type Conversion2/1 -> [cmd]
  Data Type Conversion4/1 -> [typemask]
  [mode] -> Mux/1
  [cmd] -> Mux/2
  [typemask] -> Mux/3
  coptertype/1 -> [copterType]
  [copterType] -> Mux/4
  zeros/1 -> Switch/3
  0/1 -> getMask/1(In1)
  X/1 -> getMask/2(In2)
  X1/1 -> getMask1/2(In2)
  1/1 -> getMask1/1(In1)
  2/1 -> getMask2/1(In1)
  X2/1 -> getMask2/2(In2)
  3/1 -> getMask3/1(In1)
  X3/1 -> getMask3/2(In2)
  4/1 -> getMask4/1(In1)
  X4/1 -> getMask4/2(In2)
  X5/1 -> getMask5/2(In2)
  5/1 -> getMask5/1(In1)
  X6/1 -> getMask6/2(In2)
  6/1 -> getMask6/1(In1)
  X7/1 -> getMask7/2(In2)
  7/1 -> getMask7/1(In1)
  8/1 -> getMask8/1(In1)
  X8/1 -> getMask8/2(In2)
  X9/1 -> getMask9/2(In2)
  Logical Operator/1 -> getMask9/1(In1)
  9/1 -> Logical Operator/1
  X10/1 -> getMask10/2(In2)
  10/1 -> getMask10/1(In1)
  11/1 -> getMask11/1(In1)
  X11/1 -> getMask11/2(In2)
  getMask11/1(Out1) -> Bitwise Operator1/13
  getMask10/1(Out1) -> Bitwise Operator1/12
  getMask9/1(Out1) -> Bitwise Operator1/11
  getMask8/1(Out1) -> Bitwise Operator1/10
  getMask7/1(Out1) -> Bitwise Operator1/9
  getMask6/1(Out1) -> Bitwise Operator1/8
  getMask5/1(Out1) -> Bitwise Operator1/7
  getMask4/1(Out1) -> Bitwise Operator1/6
  getMask3/1(Out1) -> Bitwise Operator1/5
  getMask2/1(Out1) -> Bitwise Operator1/4
  getMask1/1(Out1) -> Bitwise Operator1/3
  Demux2/1 -> Mux/15, Mux/12, Mux/9
  Demux2/2 -> Mux/16, Mux/13, Mux/10
  Demux2/3 -> Mux/17, Mux/14, Mux/11
  Demux2/4 -> Mux/20, Mux/23
  ZERO/1 -> Mux/22, Mux/21, Mux/28, Mux/27, Mux/26, Mux/25, Mux/24, Mux/19, Mux/18, Mux/8, Mux/7, Mux/5, Mux/6
  Switch/1 -> Demux2/1
  isEnCtrl/1 -> Switch/2
  Ctrls/1 -> Switch/1
  cmd/1 -> Bitwise Operator/1

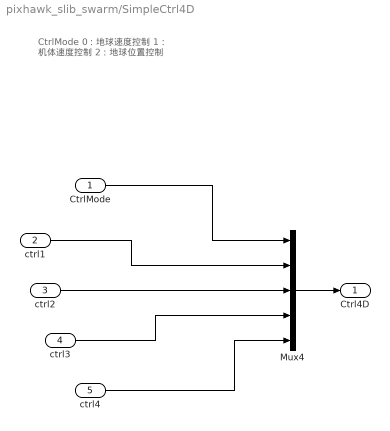
== system pixhawk_slib_swarm/SimpleCtrl4D ==
  note: CtrlMode
      | 0：地球速度控制
      | 1： 机体速度控制
      | 2：地球位置控制
  CtrlMode : Inport
  ctrl1 : Inport  Port=2
  ctrl2 : Inport  Port=3
  ctrl3 : Inport  Port=4
  ctrl4 : Inport  Port=5
  Mux4 : Mux  Inputs=5
  Ctrl4D : Outport  PortDimensions=5  VectorParamsAs1DForOutWhenUnconnected=off
  wires:
  ctrl3/1 -> Mux4/4
  ctrl2/1 -> Mux4/3
  ctrl4/1 -> Mux4/5
  ctrl1/1 -> Mux4/2
  Mux4/1 -> Ctrl4D/1
  CtrlMode/1 -> Mux4/1

== system pixhawk_slib_swarm/Simple_data_decoder ==
  simple_data : Inport  PortDimensions=12
  Bus Creator : BusCreator  Inputs=4
  Demux2 : Demux
  simple_bus : Outport  VectorParamsAs1DForOutWhenUnconnected=off
  wires:
  Bus Creator/1 -> simple_bus/1
  simple_data/1 -> Demux2/1
  Demux2/1 -> Bus Creator/1  "globalPos"
  Demux2/4 -> Bus Creator/4  "localVel"
  Demux2/2 -> Bus Creator/2  "AngEular"
  Demux2/3 -> Bus Creator/3  "localPos"

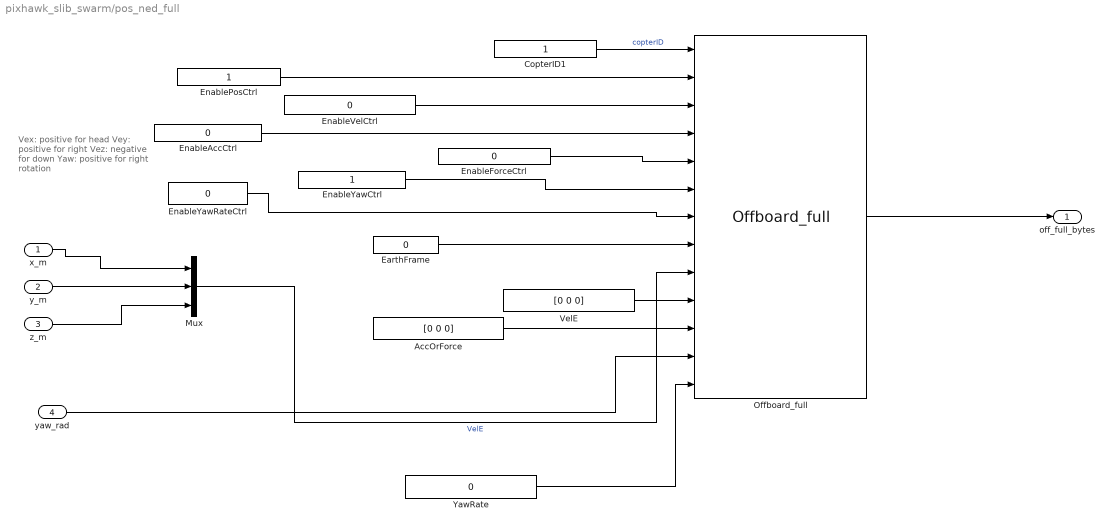
== system pixhawk_slib_swarm/pos_ned_full ==
  note: Vex: positive for head
      | Vey: positive for right
      | Vez: negative for down
      | Yaw: positive for right rotation
  x_m : Inport
  y_m : Inport  Port=2
  z_m : Inport  Port=3
  yaw_rad : Inport  Port=4  PortDimensions=1
  AccOrForce : Constant  Value=[0 0 0]
  CopterID1 : Constant
  EarthFrame : Constant  Value=0
  EnableAccCtrl : Constant  Value=0
  EnableForceCtrl : Constant  Value=0
  EnablePosCtrl : Constant
  EnableVelCtrl : Constant  Value=0
  EnableYawCtrl : Constant
  EnableYawRateCtrl : Constant  Value=0
  Mux : Mux  Inputs=3
  Offboard_full : $bdroot/Offboard_full
  VelE : Constant  Value=[0 0 0]
  YawRate : Constant  Value=0
  off_full_bytes : Outport
  wires:
  YawRate/1 -> Offboard_full/13
  EnableYawRateCtrl/1 -> Offboard_full/7
  EnableYawCtrl/1 -> Offboard_full/6
  EnableAccCtrl/1 -> Offboard_full/4
  Mux/1 -> Offboard_full/9  "VelE"
  EarthFrame/1 -> Offboard_full/8
  yaw_rad/1 -> Offboard_full/12
  AccOrForce/1 -> Offboard_full/11
  EnableVelCtrl/1 -> Offboard_full/3
  EnableForceCtrl/1 -> Offboard_full/5
  CopterID1/1 -> Offboard_full/1  "copterID"
  EnablePosCtrl/1 -> Offboard_full/2
  VelE/1 -> Offboard_full/10
  y_m/1 -> Mux/2
  x_m/1 -> Mux/1
  z_m/1 -> Mux/3
  Offboard_full/1 -> off_full_bytes/1

== system pixhawk_slib_swarm/real_data_decoder ==
  real_data : Inport
  Bus Creator : BusCreator  Inputs=27
  Decoder1 : MATLAB Function  TreatAsAtomicUnit=on
  real_bus : Outport  VectorParamsAs1DForOutWhenUnconnected=off
  wires:
  Decoder1/1(globalPos) -> Bus Creator/1  "globalPos"
  real_data/1 -> Decoder1/1(u)
  Decoder1/6(selfCheckState) -> Bus Creator/6  "selfCheckState"
  Decoder1/7(isHeartRec) -> Bus Creator/7  "isHeartRec"
  Decoder1/8(TargetSysID) -> Bus Creator/8  "TargetSysID"
  Decoder1/10(isLocalNed) -> Bus Creator/10  "isLocalNed"
  Decoder1/11(isArmed) -> Bus Creator/11  "isArmed"
  Decoder1/12(isOffboard) -> Bus Creator/12  "isOffboard"
  Decoder1/13(isFailSafeEn) -> Bus Creator/13  "isFailSafeEn"
  Decoder1/14(base_mode) -> Bus Creator/14  "base_mode"
  Decoder1/15(custom_mode) -> Bus Creator/15  "custom_mode"
  Decoder1/16(system_status) -> Bus Creator/16  "system_status"
  Decoder1/17(batteryInfo) -> Bus Creator/17  "batteryInfo"
  Decoder1/18(flyMode) -> Bus Creator/18  "flyMode"
  Decoder1/19(isStanby) -> Bus Creator/19  "isStanby"
  Decoder1/20(isActive) -> Bus Creator/20  "isActive"
  Decoder1/21(isLowBatt) -> Bus Creator/21  "isLowBatt"
  Decoder1/22(isHighLoad) -> Bus Creator/22  "isHighLoad"
  Decoder1/23(isDropComm) -> Bus Creator/23  "isDropComm"
  Decoder1/24(isGlobPos) -> Bus Creator/24  "isGlobPos"
  Decoder1/25(isGpsHome) -> Bus Creator/25  "isGpsHome"
  Bus Creator/1 -> real_bus/1
  Decoder1/5(keyPressed) -> Bus Creator/5  "keyPressed"
  Decoder1/9(TargetCompID) -> Bus Creator/9  "TargetCompID"
  Decoder1/26(isSimorExe) -> Bus Creator/26  "isSimorExe"
  Decoder1/2(AngEular) -> Bus Creator/2  "AngEular"
  Decoder1/3(localPos) -> Bus Creator/3  "localPos"
  Decoder1/4(localVel) -> Bus Creator/4  "localVel"
  Decoder1/27(obstacle) -> Bus Creator/27  "obstacle"

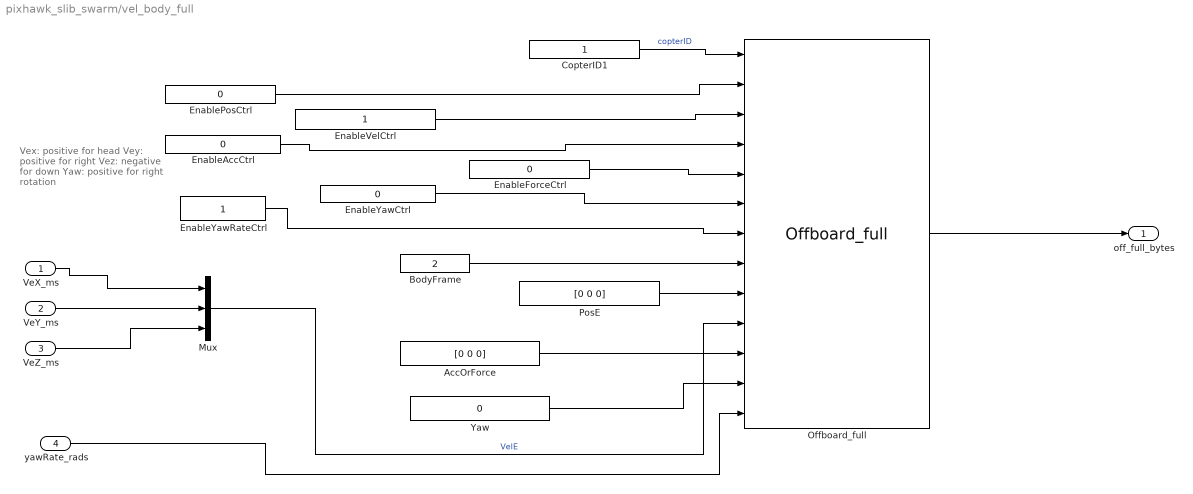
== system pixhawk_slib_swarm/vel_body_full ==
  note: Vex: positive for head
      | Vey: positive for right
      | Vez: negative for down
      | Yaw: positive for right rotation
  VeX_ms : Inport
  VeY_ms : Inport  Port=2
  VeZ_ms : Inport  Port=3
  yawRate_rads : Inport  Port=4  PortDimensions=1
  AccOrForce : Constant  Value=[0 0 0]
  BodyFrame : Constant  Value=2
  CopterID1 : Constant
  EnableAccCtrl : Constant  Value=0
  EnableForceCtrl : Constant  Value=0
  EnablePosCtrl : Constant  Value=0
  EnableVelCtrl : Constant
  EnableYawCtrl : Constant  Value=0
  EnableYawRateCtrl : Constant
  Mux : Mux  Inputs=3
  Offboard_full : $bdroot/Offboard_full
  PosE : Constant  Value=[0 0 0]
  Yaw : Constant  Value=0
  off_full_bytes : Outport
  wires:
  Yaw/1 -> Offboard_full/12
  EnableYawRateCtrl/1 -> Offboard_full/7
  EnableYawCtrl/1 -> Offboard_full/6
  EnableAccCtrl/1 -> Offboard_full/4
  Mux/1 -> Offboard_full/10  "VelE"
  BodyFrame/1 -> Offboard_full/8
  yawRate_rads/1 -> Offboard_full/13
  AccOrForce/1 -> Offboard_full/11
  EnableVelCtrl/1 -> Offboard_full/3
  EnableForceCtrl/1 -> Offboard_full/5
  CopterID1/1 -> Offboard_full/1  "copterID"
  EnablePosCtrl/1 -> Offboard_full/2
  PosE/1 -> Offboard_full/9
  VeY_ms/1 -> Mux/2
  VeX_ms/1 -> Mux/1
  VeZ_ms/1 -> Mux/3
  Offboard_full/1 -> off_full_bytes/1

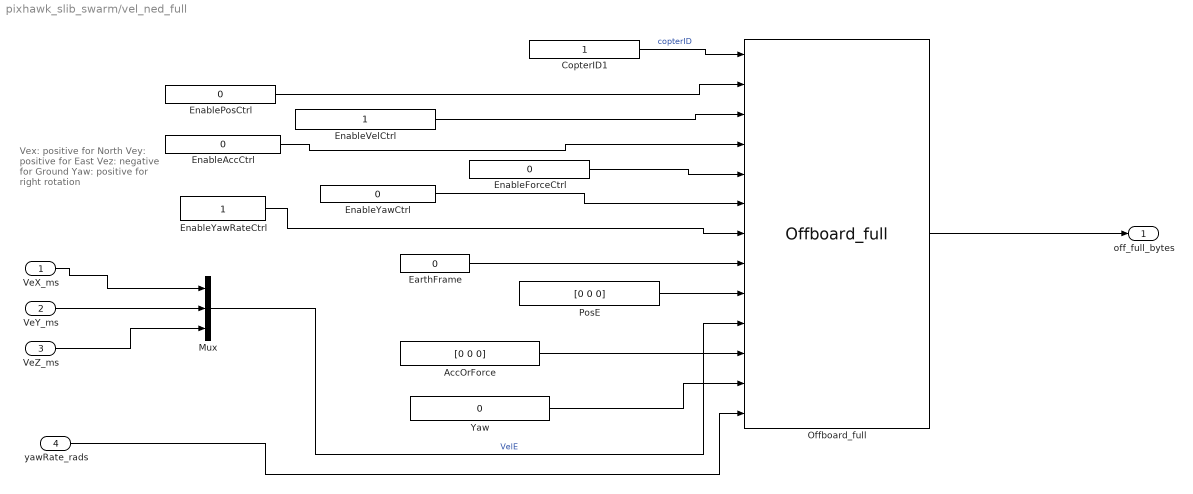
== system pixhawk_slib_swarm/vel_ned_full ==
  note: Vex: positive for North
      | Vey: positive for East
      | Vez: negative for Ground
      | Yaw: positive for right rotation
  VeX_ms : Inport
  VeY_ms : Inport  Port=2
  VeZ_ms : Inport  Port=3
  yawRate_rads : Inport  Port=4  PortDimensions=1
  AccOrForce : Constant  Value=[0 0 0]
  CopterID1 : Constant
  EarthFrame : Constant  Value=0
  EnableAccCtrl : Constant  Value=0
  EnableForceCtrl : Constant  Value=0
  EnablePosCtrl : Constant  Value=0
  EnableVelCtrl : Constant
  EnableYawCtrl : Constant  Value=0
  EnableYawRateCtrl : Constant
  Mux : Mux  Inputs=3
  Offboard_full : $bdroot/Offboard_full
  PosE : Constant  Value=[0 0 0]
  Yaw : Constant  Value=0
  off_full_bytes : Outport
  wires:
  Yaw/1 -> Offboard_full/12
  EnableYawRateCtrl/1 -> Offboard_full/7
  EnableYawCtrl/1 -> Offboard_full/6
  EnableAccCtrl/1 -> Offboard_full/4
  Mux/1 -> Offboard_full/10  "VelE"
  EarthFrame/1 -> Offboard_full/8
  yawRate_rads/1 -> Offboard_full/13
  AccOrForce/1 -> Offboard_full/11
  EnableVelCtrl/1 -> Offboard_full/3
  EnableForceCtrl/1 -> Offboard_full/5
  CopterID1/1 -> Offboard_full/1  "copterID"
  EnablePosCtrl/1 -> Offboard_full/2
  PosE/1 -> Offboard_full/9
  VeY_ms/1 -> Mux/2
  VeX_ms/1 -> Mux/1
  VeZ_ms/1 -> Mux/3
  Offboard_full/1 -> off_full_bytes/1

== system pixhawk_slib_swarm/vrpn_data_decoder ==
  vrpn_data : Inport
  Bus Creator : BusCreator  Inputs=10
  Decoder : MATLAB Function  TreatAsAtomicUnit=on
  vrpn_bus : Outport  VectorParamsAs1DForOutWhenUnconnected=off
  wires:
  vrpn_data/1 -> Decoder/1(u)
  Bus Creator/1 -> vrpn_bus/1
  Decoder/1(t_pos) -> Bus Creator/1  "t_pos"
  Decoder/2(pos_xyz) -> Bus Creator/2  "pos"
  Decoder/3(quat_wxyz) -> Bus Creator/3  "quat_wxyz"
  Decoder/4(euler) -> Bus Creator/4  "euler"
  Decoder/5(t_vel) -> Bus Creator/5  "t_vel"
  Decoder/6(vel_xyz) -> Bus Creator/6  "v"
  Decoder/7(t_acc) -> Bus Creator/7  "t_acc"
  Decoder/8(acc_xyz) -> Bus Creator/8  "acc"
  Decoder/9(has_data) -> Bus Creator/9  "has_data"
  Decoder/10(has_pos) -> Bus Creator/10  "has_pos"

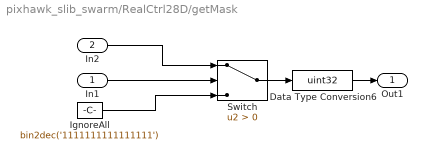
== system pixhawk_slib_swarm/RealCtrl28D/getMask ==
  In1 : Inport
  In2 : Inport  Port=2
  Data Type Conversion6 : DataTypeConversion  OutDataTypeStr=uint32  SaturateOnIntegerOverflow=off  RndMeth=Floor
  IgnoreAll : Constant  Value=bin2dec('1111111111111111')
  Switch : Switch  Criteria=u2 > Threshold  SaturateOnIntegerOverflow=off  InputSameDT=off
  Out1 : Outport  VectorParamsAs1DForOutWhenUnconnected=off
  wires:
  In1/1 -> Switch/2
  Switch/1 -> Data Type Conversion6/1
  Data Type Conversion6/1 -> Out1/1
  IgnoreAll/1 -> Switch/3
  In2/1 -> Switch/1

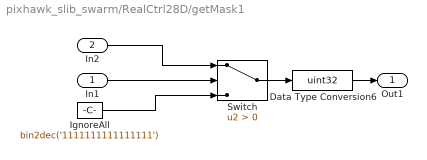
== system pixhawk_slib_swarm/RealCtrl28D/getMask1 ==
  In1 : Inport
  In2 : Inport  Port=2
  Data Type Conversion6 : DataTypeConversion  OutDataTypeStr=uint32  SaturateOnIntegerOverflow=off  RndMeth=Floor
  IgnoreAll : Constant  Value=bin2dec('1111111111111111')
  Switch : Switch  Criteria=u2 > Threshold  SaturateOnIntegerOverflow=off  InputSameDT=off
  Out1 : Outport  VectorParamsAs1DForOutWhenUnconnected=off
  wires:
  In1/1 -> Switch/2
  Switch/1 -> Data Type Conversion6/1
  Data Type Conversion6/1 -> Out1/1
  IgnoreAll/1 -> Switch/3
  In2/1 -> Switch/1

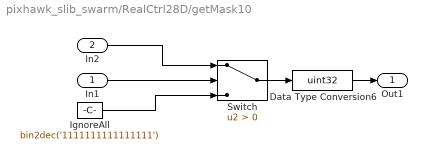
== system pixhawk_slib_swarm/RealCtrl28D/getMask10 ==
  In1 : Inport
  In2 : Inport  Port=2
  Data Type Conversion6 : DataTypeConversion  OutDataTypeStr=uint32  SaturateOnIntegerOverflow=off  RndMeth=Floor
  IgnoreAll : Constant  Value=bin2dec('1111111111111111')
  Switch : Switch  Criteria=u2 > Threshold  SaturateOnIntegerOverflow=off  InputSameDT=off
  Out1 : Outport  VectorParamsAs1DForOutWhenUnconnected=off
  wires:
  In1/1 -> Switch/2
  Switch/1 -> Data Type Conversion6/1
  Data Type Conversion6/1 -> Out1/1
  IgnoreAll/1 -> Switch/3
  In2/1 -> Switch/1

== system pixhawk_slib_swarm/RealCtrl28D/getMask11 ==
  In1 : Inport
  In2 : Inport  Port=2
  Data Type Conversion6 : DataTypeConversion  OutDataTypeStr=uint32  SaturateOnIntegerOverflow=off  RndMeth=Floor
  IgnoreAll : Constant  Value=bin2dec('1111111111111111')
  Switch : Switch  Criteria=u2 > Threshold  SaturateOnIntegerOverflow=off  InputSameDT=off
  Out1 : Outport  VectorParamsAs1DForOutWhenUnconnected=off
  wires:
  In1/1 -> Switch/2
  Switch/1 -> Data Type Conversion6/1
  Data Type Conversion6/1 -> Out1/1
  IgnoreAll/1 -> Switch/3
  In2/1 -> Switch/1

== system pixhawk_slib_swarm/RealCtrl28D/getMask2 ==
  In1 : Inport
  In2 : Inport  Port=2
  Data Type Conversion6 : DataTypeConversion  OutDataTypeStr=uint32  SaturateOnIntegerOverflow=off  RndMeth=Floor
  IgnoreAll : Constant  Value=bin2dec('1111111111111111')
  Switch : Switch  Criteria=u2 > Threshold  SaturateOnIntegerOverflow=off  InputSameDT=off
  Out1 : Outport  VectorParamsAs1DForOutWhenUnconnected=off
  wires:
  In1/1 -> Switch/2
  Switch/1 -> Data Type Conversion6/1
  Data Type Conversion6/1 -> Out1/1
  IgnoreAll/1 -> Switch/3
  In2/1 -> Switch/1

== system pixhawk_slib_swarm/RealCtrl28D/getMask3 ==
  In1 : Inport
  In2 : Inport  Port=2
  Data Type Conversion6 : DataTypeConversion  OutDataTypeStr=uint32  SaturateOnIntegerOverflow=off  RndMeth=Floor
  IgnoreAll : Constant  Value=bin2dec('1111111111111111')
  Switch : Switch  Criteria=u2 > Threshold  SaturateOnIntegerOverflow=off  InputSameDT=off
  Out1 : Outport  VectorParamsAs1DForOutWhenUnconnected=off
  wires:
  In1/1 -> Switch/2
  Switch/1 -> Data Type Conversion6/1
  Data Type Conversion6/1 -> Out1/1
  IgnoreAll/1 -> Switch/3
  In2/1 -> Switch/1

== system pixhawk_slib_swarm/RealCtrl28D/getMask4 ==
  In1 : Inport
  In2 : Inport  Port=2
  Data Type Conversion6 : DataTypeConversion  OutDataTypeStr=uint32  SaturateOnIntegerOverflow=off  RndMeth=Floor
  IgnoreAll : Constant  Value=bin2dec('1111111111111111')
  Switch : Switch  Criteria=u2 > Threshold  SaturateOnIntegerOverflow=off  InputSameDT=off
  Out1 : Outport  VectorParamsAs1DForOutWhenUnconnected=off
  wires:
  In1/1 -> Switch/2
  Switch/1 -> Data Type Conversion6/1
  Data Type Conversion6/1 -> Out1/1
  IgnoreAll/1 -> Switch/3
  In2/1 -> Switch/1

== system pixhawk_slib_swarm/RealCtrl28D/getMask5 ==
  In1 : Inport
  In2 : Inport  Port=2
  Data Type Conversion6 : DataTypeConversion  OutDataTypeStr=uint32  SaturateOnIntegerOverflow=off  RndMeth=Floor
  IgnoreAll : Constant  Value=bin2dec('1111111111111111')
  Switch : Switch  Criteria=u2 > Threshold  SaturateOnIntegerOverflow=off  InputSameDT=off
  Out1 : Outport  VectorParamsAs1DForOutWhenUnconnected=off
  wires:
  In1/1 -> Switch/2
  Switch/1 -> Data Type Conversion6/1
  Data Type Conversion6/1 -> Out1/1
  IgnoreAll/1 -> Switch/3
  In2/1 -> Switch/1
